simulink model "PSO_PID_dif_Frecuencia"  (R2025a)
settings: Solver=FixedStepAuto  StartTime=0.0  StopTime=19  FixedStep=0.01  RelTol=1e-3
undefined symbols (not defined in the file or in its folder): CR, DiscIntNeverNeededParam, K_fd, K_fi, K_fp, LF
libraries: instrumentseriallib x3, simulink x1
settings Model: Creator=jorge  LastModifiedBy=sergio2416

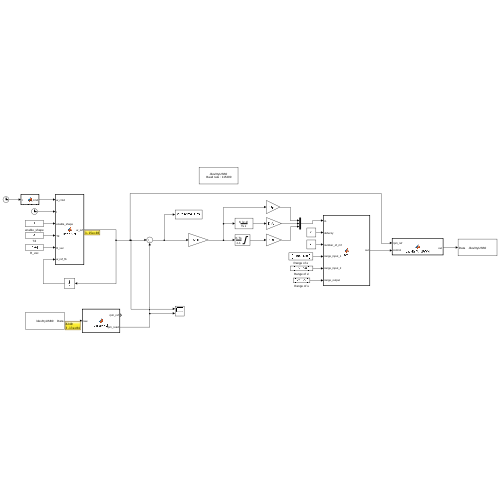
[thumbnail: Simulink's stored preview of the top-level diagram]
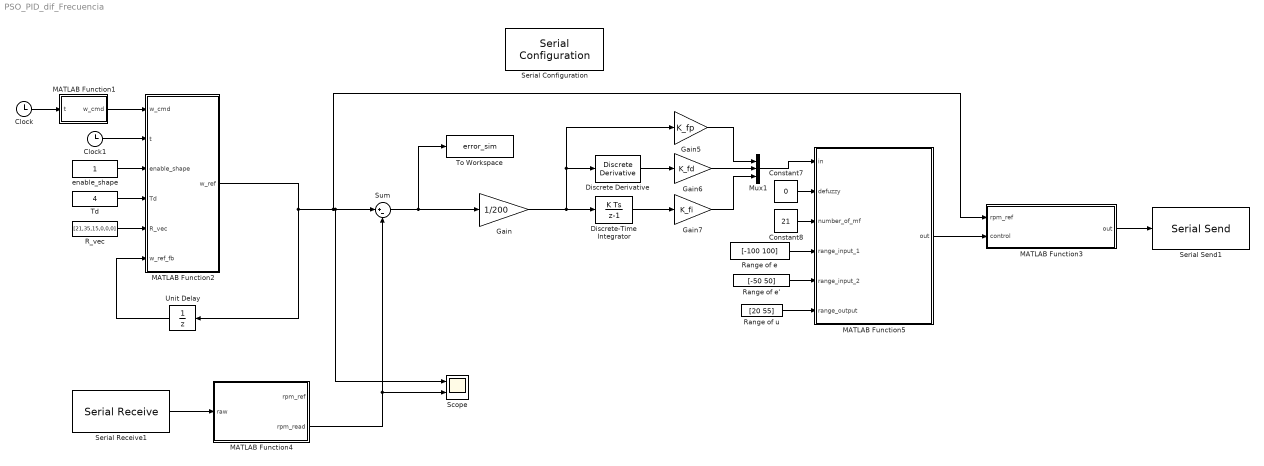
== system PSO_PID_dif_Frecuencia ==
  Clock : Clock
  Clock1 : Clock
  Constant7 : Constant  Value=0
  Constant8 : Constant  Value=21
  Discrete Derivative : simulink/Discrete/Discrete Derivative  gainval=1.0  ICPrevScaledInput=0.0  OutMin=[]  OutMax=[]  OutDataType=fixdt(1, 16)  OutScaling=2^-10  DoSatur=off
  Discrete-Time Integrator : DiscreteIntegrator  SampleTime=0.01  LimitOutput=on  UpperSaturationLimit=65  LowerSaturationLimit=0  ICPrevOutput=DiscIntNeverNeededParam  ICPrevScaledInput=DiscIntNeverNeededParam
  Gain : Gain  Gain=1/200
  Gain5 : Gain  Gain=K_fp
  Gain6 : Gain  Gain=K_fd
  Gain7 : Gain  Gain=K_fi
  MATLAB Function1 : MATLAB Function  TreatAsAtomicUnit=on
  MATLAB Function2 : MATLAB Function  TreatAsAtomicUnit=on
  MATLAB Function3 : MATLAB Function  TreatAsAtomicUnit=on
  MATLAB Function4 : MATLAB Function  TreatAsAtomicUnit=on
  MATLAB Function5 : MATLAB Function  TreatAsAtomicUnit=on
  Mux1 : Mux  Inputs=3
  R_vec : Constant  Value=[21,35,15,0,0,0]  SampleTime=-1
  Range of e : Constant  Value=[-100 100]
  Range of e' : Constant  Value=[-50 50]
  Range of u : Constant  Value=[20 55]
  Scope : Scope  NumInputPorts=2
      settings: ActiveDisplayYMinimum=-3270.6249999999991  ActiveDisplayYMaximum=35145.625
  Serial Configuration : instrumentseriallib/Serial Configuration  Priority=-200000  PortSel=/dev/ttyUSB0  Port=/dev/ttyUSB0  ComPort=/dev/ttyUSB0  BaudRate=115200  DataBits=8  Parity=none  StopBits=1  ByteOrder=little-endian  FlowControl=none  Timeout=10  SimulateUsing=Interpreted execution  BlockInModel=on  aMode=1
  Serial Receive1 : instrumentseriallib/Serial Receive  Priority=1  PortSel=/dev/ttyUSB0  Port=/dev/ttyUSB0  ComPort=/dev/ttyUSB0  DataType=int16  SaveDataType=uint8  ToggleHeader=off  Header=[]  ToggleDataSize=on  DataSize=[2 1]  ToggleTerminator=off  Terminator=CR/LF ('\r\n')  CustomTerminator=[]  InputFormat=Column major  EnableBlockingMode=on  ActionDataUnavailable=Output last received value  ActionWhenDataUnavailable=Output last received value  CustomValue=0  SampleTime=0.01  SimulateUsing=Interpreted execution  BlockInModel=on  aMode=1  LibraryInUse=instrumentlib
  Serial Send1 : instrumentseriallib/Serial Send  Priority=1  PortSel=/dev/ttyUSB0  Port=/dev/ttyUSB0  ComPort=/dev/ttyUSB0  Header=[]  Terminator=<none>  CustomTerminator=[]  EnableBlockingMode=off  SimulateUsing=Interpreted execution  BlockInModel=on  aMode=1
  Sum : Sum  Inputs=|+-
  Td : Constant  Value=4  SampleTime=-1
  To Workspace : ToWorkspace  VariableName=error_sim  SampleTime=-1
      settings: Save2DSignal=2-D array (concatenate along first dimension)
  Unit Delay : UnitDelay  SampleTime=-1  HasFrameUpgradeWarning=on
  enable_shape : Constant  SampleTime=-1
  wires:
  Clock/1 -> MATLAB Function1/1(t)
  Clock1/1 -> MATLAB Function2/2(t)
  MATLAB Function2/1(w_ref) -> MATLAB Function3/1(rpm_ref), Scope/1, Sum/1, Unit Delay/1
  enable_shape/1 -> MATLAB Function2/3(enable_shape)
  Td/1 -> MATLAB Function2/4(Td)
  MATLAB Function1/1(w_cmd) -> MATLAB Function2/1(w_cmd)
  R_vec/1 -> MATLAB Function2/5(R_vec)
  Unit Delay/1 -> MATLAB Function2/6(w_ref_fb)
  Range of u/1 -> MATLAB Function5/6(range_output)
  Discrete Derivative/1 -> Gain6/1
  Constant8/1 -> MATLAB Function5/3(number_of_mf)
  Gain5/1 -> Mux1/1
  Range of e/1 -> MATLAB Function5/4(range_input_1)
  Gain7/1 -> Mux1/3
  Mux1/1 -> MATLAB Function5/1(in)
  Range of e'/1 -> MATLAB Function5/5(range_input_2)
  Sum/1 -> Gain/1, To Workspace/1
  Gain6/1 -> Mux1/2
  Discrete-Time Integrator/1 -> Gain7/1
  Constant7/1 -> MATLAB Function5/2(defuzzy)
  Gain/1 -> Gain5/1, Discrete Derivative/1, Discrete-Time Integrator/1
  MATLAB Function3/1(out) -> Serial Send1/1
  MATLAB Function5/1(out) -> MATLAB Function3/2(control)
  Serial Receive1/1 -> MATLAB Function4/1(raw)
  MATLAB Function4/2(rpm_read) -> Scope/2, Sum/2

== matlab function PSO_PID_dif_Frecuencia/MATLAB Function1 ==
  data: t input; w_cmd output
function w_cmd = Generador_Perfil(t)
    % Genera la señal escalón para alimentar al suavizador Bezier
    % Secuencia: 540 -> 1160 -> 800
    
    % --- CONFIGURACIÓN DE TIEMPOS ---
    % Td es 4 segundos. Dejamos un margen para que se estabilice.
    t_inicio = 4;   % Tiempo para el primer cambio (540 -> 1160)
    t_bajada = 13;  % Tiempo para el segundo cambio (1160 -> 800)
    
    % --- LÓGICA DE COMANDO ---
    if t < t_inicio
        % Estado inicial
        w_cmd = 600;
        
    elseif t >= t_inicio && t < t_bajada
        % Primer escalón: Subida
        w_cmd = 1160;
        
    else
        % Segundo escalón: Bajada
        w_cmd = 800;
    end
end

== matlab function PSO_PID_dif_Frecuencia/MATLAB Function2 ==
  settings: updateMethod=DISCRETE
  data: w_cmd input; t input; w_ref output; enable_shape input; Td input; R_vec input; w_ref_fb input
function w_ref = BezierRef(w_cmd, t, enable_shape, Td, R_vec, w_ref_fb)
% =================================================================
% VERSIÓN 6 (Corrección de arranque en cero)
% =================================================================
%
% Entradas:
%   w_cmd     : setpoint deseado (de la GUI)
%   t         : tiempo absoluto (Clock)
%   enable_shape : 1 = perfilar, 0 = paso directo
%   Td        : duración de la transición [s]
%   R_vec     : [r1..r6] coeficientes del polinomio
%   w_ref_fb  : w_ref anterior (feedback vía Memory/Unit Delay)
%
% Salida:
%   w_ref     : referencia suavizada

% --- estados persistentes ---
persistent w0 wf t0 last_cmd is_initialized

% --- Lógica de inicialización en el primer paso de ejecución ---
if isempty(is_initialized) || t == 0 % Se reinicia si el tiempo es 0
    is_initialized = true; 
    
    % --- CORRECCIÓN AQUÍ ---
    % Antes decía: w0 = w_ref_fb; (Esto tomaba el 0 del Unit Delay)
    % Ahora dice:
    w0 = w_cmd;  % Forzamos a que el punto de partida sea el comando actual (540)
    wf = w_cmd;
    
    t0 = t;
    last_cmd = w_cmd;
end

% --- FIX 1: Detecta cambio de comando con tolerancia ---
if abs(w_cmd - last_cmd) > 1e-6
    % AQUÍ SÍ usamos w_ref_fb, porque queremos una curva suave desde
    % donde nos quedamos anteriormente.
    w0 = w_ref_fb;
    wf = w_cmd;
    t0 = t;
    last_cmd = w_cmd;
end

% Paso directo si está desactivado
if enable_shape == 0 || Td <= 0
    w_ref = w_cmd;
    w0 = w_cmd; 
    wf = w_cmd;
    last_cmd = w_cmd;
    return
end

% Progreso normalizado en [0,1]
s = (t - t0) / Td;

if s <= 0
    alpha = 0;
elseif s >= 1
    alpha = 1;
else
    % Bezier polinómico
    if numel(R_vec) < 6
        alpha = s; % Fallback a rampa lineal
    else
        r1 = R_vec(1); r2 = R_vec(2); r3 = R_vec(3);
        r4 = R_vec(4); r5 = R_vec(5); r6 = R_vec(6);
        
        % Validación de coeficientes
        if abs((r1 - r2 + r3 - r4 + r5 - r6) - 1.0) > 1e-3
            alpha = s^5;
        else
            alpha = (s.^5).*(r1 - r2*s + r3*s.^2 - r4*s.^3 + r5*s.^4 - r6*s.^5);
        end
    end
    
    % Clampeo por seguridad numérica
    if alpha < 0, alpha = 0; end
    if alpha > 1, alpha = 1; end
end

% Interpolación entre w0 y wf
w_ref = w0 + alpha*(wf - w0);
end

== matlab function PSO_PID_dif_Frecuencia/MATLAB Function4 ==
  data: rpm_ref output; rpm_read output; raw input
function [rpm_ref, rpm_read] = parseRPM(raw)
%#codegen
% raw: 1x2 uint16 vector received from ESP32
% rpm_read: measured RPM from encoder
% rpm_ref:  reference RPM echoed back from ESP32

rpm_read = double(raw(2));   % first  uint16 from ESP32
rpm_ref  = double(raw(1));   % second uint16 from ESP32
end

== matlab function PSO_PID_dif_Frecuencia/MATLAB Function5 ==
  data: in input; out output; defuzzy input; number_of_mf input; range_input_1 input; range_input_2 input; range_output input
function out = fcn(in, defuzzy, number_of_mf, range_input_1, range_input_2, range_output)
% ------------------------------------------------------------
%   Fuzzy PD compacto (discreto)
%   Entradas:
%     in(1) = error
%     in(2) = derror
%
%   NOTA: Ignoramos los parámetros externos y usamos
%         valores internos estables optimizados
% ------------------------------------------------------------

    % -------- Configuración FIS --------
    number_of_mf = 21;

    % Rango de error sugerido
    range_input_1_min = -250;
    range_input_1_max = 250;

    % Rango de d(error)
    range_input_2_min = -120;
    range_input_2_max = 120;

    % Rango de salida
    range_output_min = 20;
    range_output_max = 55;

    % Bias centrado en el rango de salida
    output_bias = (range_output_min + range_output_max) / 2;     % 37.5

    % Ganancia para hacer más sensible la salida fuzzy
    fuzzy_gain = 2.0;

    % ---------------------------------------------------------

    % Entradas
    error  = in(1);
    derror = in(2);

    % Saturar error
    error = max(min(error,  range_input_1_max), range_input_1_min);
    derror = max(min(derror, range_input_2_max), range_input_2_min);

    % Paso entre funciones de membresía
    step_e  = (range_input_1_max - range_input_1_min) / (number_of_mf - 1);
    step_de = (range_input_2_max - range_input_2_min) / (number_of_mf - 1);

    % Índices difusos
    idx_e  = floor((error  - range_input_1_min) / step_e);
    idx_de = floor((derror - range_input_2_min) / step_de);

    % Limitar índices
    idx_e  = max(min(idx_e,  number_of_mf - 1), 0);
    idx_de = max(min(idx_de, number_of_mf - 1), 0);

    % Regla PD difusa
    fuzzy_index = idx_e + idx_de - floor(number_of_mf/2);

    % Limitar fuzzy_index
    fuzzy_index = max(min(fuzzy_index, 10), -10);

    % Salida fuzzy normalizada [-1,1]
    fuzzy_pd_out = fuzzy_index / 10;

    % Ganancia
    fuzzy_pd_out = fuzzy_pd_out * fuzzy_gain;

    % Duty
    duty = output_bias + fuzzy_pd_out * 10;

    % Saturar duty
    duty = max(min(duty, range_output_max), range_output_min);

    % Salida
    out = duty;
end

== matlab function PSO_PID_dif_Frecuencia/MATLAB Function3 ==
  data: rpm_ref input; control input; out output
function out = packRefAndPWM(rpm_ref, control)
% Esta función ahora empaqueta [rpm_ref, frequency_hz]
% El 'control_signal' (antes 'voltage') viene de 0-60 desde el "Knob".

% --- 1. Escalado lineal ---
% Frecuencia (0-60 Hz)
target_freq = control;

% --- 2. Empaquetado ---
% Convierte ambos valores a uint16 para enviar por UART
freq_u16 = uint16(target_freq);
rpm_ref_u16 = uint16(rpm_ref);

% El ESP32 espera recibir: [rpm_ref, frecuencia_en_hz]
out = uint16([rpm_ref_u16, freq_u16]);

end
